simulink model "YXdzy"  (R2021b)
settings: Solver=VariableStepAuto  StartTime=0.0  StopTime=0.0004874439326  RelTol=1e-3
settings Model: Creator=zhonghuatu  LastModifiedBy=zhonghuatu

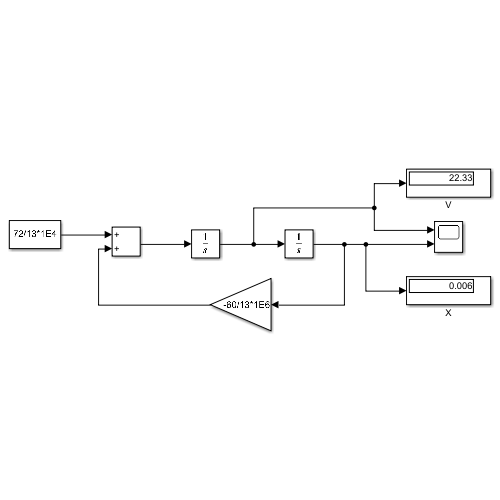
[thumbnail: Simulink's stored preview of the top-level diagram]
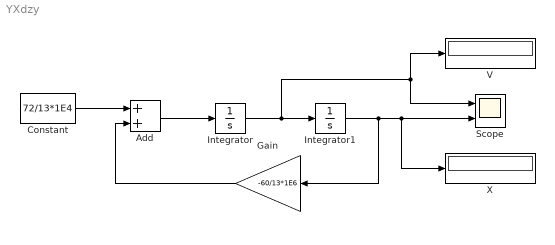
== system YXdzy ==
  Add : Sum
  Constant : Constant  Value=72/13*1E4
  Gain : Gain  Gain=-60/13*1E6
  Integrator : Integrator
  Integrator1 : Integrator
  Scope : Scope  NumInputPorts=2
  V : Display
  X : Display
  wires:
  Integrator/1 -> Scope/1, V/1, Integrator1/1
  Integrator1/1 -> X/1, Scope/2, Gain/1
  Constant/1 -> Add/1
  Gain/1 -> Add/2
  Add/1 -> Integrator/1
